simulink model "mcb_param_est_host"  (R2023a)
settings: Solver=FixedStepDiscrete  StartTime=0.0  StopTime=inf  RelTol=1e-3  EnableMultiTasking=on
undefined symbols (not defined in the file): Ts_uart
libraries: instrumentseriallib x3, embeddedblockslib x1, simulink x1
settings Model: Creator=The MathWorks, Inc.  LastModifiedBy=snarayan
settings SolverCC: AlgebraicLoopSolver=TrustRegion
settings DataIOCC: LimitDataPoints=on  SaveFormat=Array  ReturnWorkspaceOutputs=off
settings OptimizationCC: LifeSpan=1  EfficientTunableParamExpr=on
settings DebuggingCC: MergeDetectMultiDrivingBlocksExec=none  SolverPrmCheckMsg=warning  ParameterPrecisionLossMsg=none  UnconnectedInputMsg=warning  UnconnectedOutputMsg=warning  UnconnectedLineMsg=warning  AllowSymbolicDim=off  PregeneratedLibrarySubsystemCodeDiagnostic=none  SFUnexpectedBacktrackingDiag=warning  SFNoUnconditionalDefaultTransitionDiag=warning  SFExecutionAtInitializationDiag=none  ArithmeticOperatorsInVariantConditions=warning
settings HardwareCC: ProdBitPerPointer=32  ProdLargestAtomicFloat=None  ProdIntDivRoundTo=Undefined  ProdEndianess=Unspecified  ProdWordSize=32  ProdHWDeviceType=32-bit Generic
settings ModelReferenceCC: EnableRefExpFcnMdlSchedulingChecks=on  PropagateSignalLabelsOutOfModel=off
settings SFSimCC: SimUseLocalCustomCode=off  MATLABDynamicMemAlloc=off
settings RTWCC: Description=Real-Time Workshop Embedded Coder  SystemTargetFile=ert.tlc  TemplateMakefile=ert_default_tmf  GenerateReport=on  RTWUseLocalCustomCode=off  IncludeHyperlinkInReport=on  LaunchReport=on  GenerateTraceInfo=on  GenerateTraceReport=on  GenerateTraceReportSl=on  GenerateTraceReportSf=on  GenerateTraceReportEml=on  DLArmComputeVersion=19.05
settings CodeAppCC: IgnoreCustomStorageClasses=off  StateflowObjectComments=on  InternalIdentifier=Classic
settings ERTTargetCC: MultiwordLength=2048  GenerateSampleERTMain=on  ERTCustomFileTemplate=example_file_process.tlc  ConvertIfToSwitch=off  SuppressUnreachableDefaultCases=off
settings ConfigComp: CovMetricSettings=dw  CovSaveCumulativeToWorkspaceVar=on  CovSaveSingleToWorkspaceVar=on  CovExternalEMLEnable=off  CovSFcnEnable=off

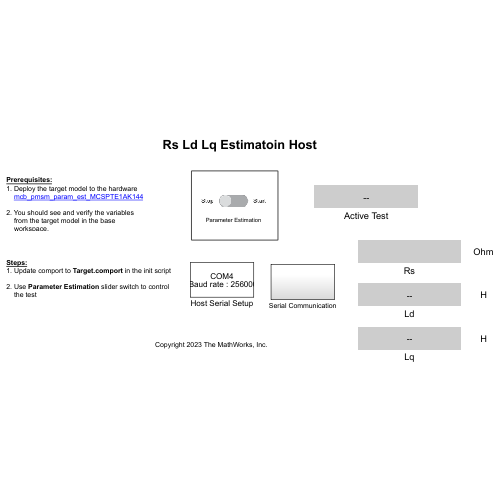
[thumbnail: Simulink's stored preview of the top-level diagram]
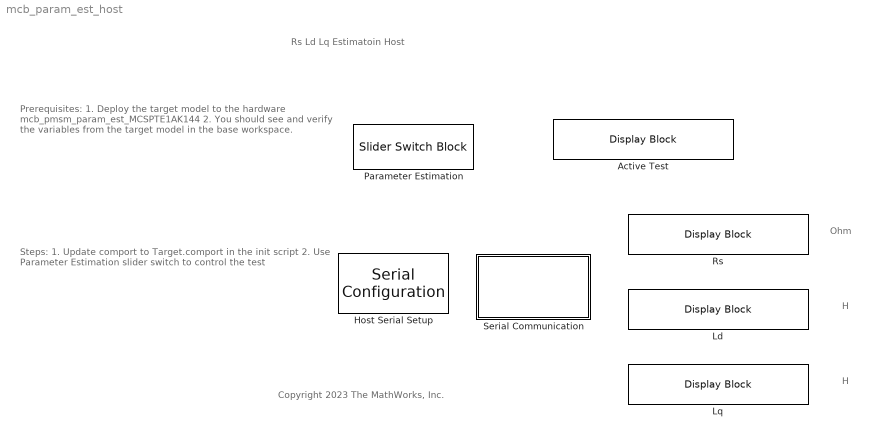
== system mcb_param_est_host ==
  note: Rs Ld Lq Estimatoin Host
  note: Copyright 2023 The MathWorks, Inc.
  note: Ohm
  note: H
  note: H
  note: Prerequisites:
      | 1. Deploy the target model to the hardware
      | mcb_pmsm_param_est_MCSPTE1AK144
      |
      | 2. You should see and verify the variables
      | from the target model in the base
      | workspace.
  note: Steps:
      | 1. Update comport to Target.comport in the init script
      |
      | 2. Use Parameter Estimation slider switch to control
      | the test
  Active Test : DisplayBlock  LabelPosition=Hide  Transparency=1
  Host Serial Setup : instrumentseriallib/Serial Configuration  Priority=-99  PortSel=Target.comport  Port=Target.comport  ComPort=Target.comport  BaudRate=256000  DataBits=8  Parity=none  StopBits=1  ByteOrder=little-endian  FlowControl=none  Timeout=2  SimulateUsing=Interpreted execution  BlockInModel=on  aMode=5
      settings: LibrarySourceBlock=mcbhostblockslib/Host Serial Setup
  Ld : DisplayBlock  LabelPosition=Hide  Transparency=1
  Lq : DisplayBlock  LabelPosition=Hide  Transparency=1
  Parameter Estimation : SliderSwitchBlock  LabelPosition=Hide
      settings: Values={{'Stop', 'Start'}, [0 1]}
  Rs : DisplayBlock  LabelPosition=Hide  Transparency=1
  Serial Communication : Subsystem

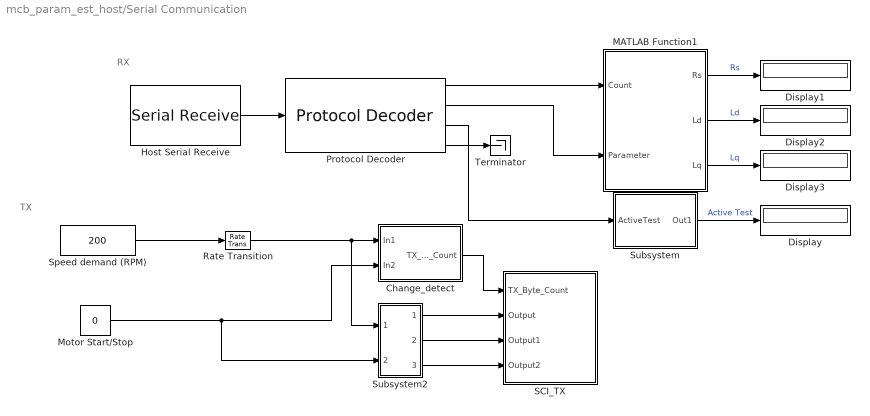
== system mcb_param_est_host/Serial Communication ==
  note: RX
  note: TX
  Change_detect : Subsystem
  Display{,1..3} (4 alike) : Display
  Host Serial Receive : instrumentseriallib/Serial Receive  PortSel=Target.comport  Port=Target.comport  ComPort=Target.comport  DataType=uint8  SaveDataType=uint8  ToggleHeader=off  Header='S'  ToggleTerminator=off  Terminator=Custom terminator  CustomTerminator='E'  InputFormat=Row major  ToggleDataSize=on  DataSize=7  EnableBlockingMode=on  ActionDataUnavailable=Output custom value  ActionWhenDataUnavailable=Output custom value  CustomValue=15  SampleTime=Ts_uart  SimulateUsing=Interpreted execution  BlockInModel=on  aMode=5
      settings: LibrarySourceBlock=mcbhostblockslib/Host Serial Receive
  MATLAB Function1 : MATLAB Function  TreatAsAtomicUnit=on
  Motor Start/Stop : Constant  Value=0  OutDataTypeStr=Inherit: Inherit via back propagation
  Protocol Decoder : embeddedblockslib/Protocol Decoder  IsParseCSV=off  Header='S'  FieldTable={ 'Count', '1', 'uint8', 'Little endian'; 'Parameter', '1', 'single', 'Little endian'; 'Active Test', '1', 'uint8', 'Little endian' }  IsVariableSizeLastField=off  MaxVariableSizeFieldLength=[]  IsChecksumRequired=off  ChecksumAlgorithm=XOR of bytes  ChecksumSize=[]  TerminatorOption=<none>  CustomTerminatorVal=[]  IsInputLengthAvailable=off
      settings: LibrarySourceBlock=c2000lib/Target Communication/Protocol Decoder
  Rate Transition : RateTransition  OutPortSampleTime=Ts_uart
  SCI_TX : Subsystem  TreatAsAtomicUnit=on
  Speed demand (RPM) : Constant  Value=200  VectorParams1D=off  OutDataTypeStr=int16  SampleTime=0.03
  Subsystem : Subsystem
  Subsystem2 : Subsystem
  Terminator : Terminator
  wires:
  Motor Start/Stop/1 -> Subsystem2/2(In2), Change_detect/2(In2)
  Rate Transition/1 -> Subsystem2/1(In1), Change_detect/1(In1)
  Speed demand (RPM)/1 -> Rate Transition/1
  Subsystem2/1(Output) -> SCI_TX/2(Output)
  Subsystem2/2(Output1) -> SCI_TX/3(Output1)
  Subsystem2/3(Output2) -> SCI_TX/4(Output2)
  Change_detect/1(TX_Byte_Count) -> SCI_TX/1(TX_Byte_Count)
  Host Serial Receive/1 -> Protocol Decoder/1
  Protocol Decoder/4 -> Terminator/1
  Protocol Decoder/2 -> MATLAB Function1/2(Parameter)
  MATLAB Function1/1(Rs) -> Display1/1  "Rs"
  MATLAB Function1/2(Ld) -> Display2/1  "Ld"
  MATLAB Function1/3(Lq) -> Display3/1  "Lq"
  Protocol Decoder/1 -> MATLAB Function1/1(Count)
  Protocol Decoder/3 -> Subsystem/1(ActiveTest)
  Subsystem/1(Out1) -> Display/1  "Active Test"

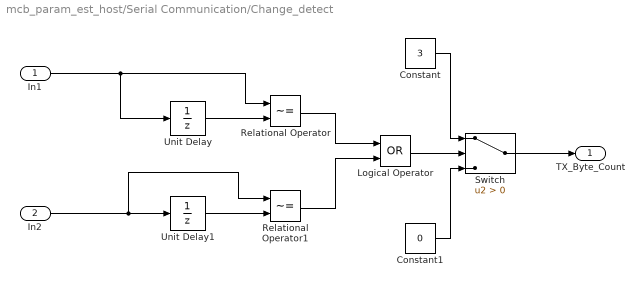
== system mcb_param_est_host/Serial Communication/Change_detect ==
  In1 : Inport
  In2 : Inport  Port=2
  Constant : Constant  Value=3  OutDataTypeStr=uint8
  Constant1 : Constant  Value=0  OutDataTypeStr=uint8
  Logical Operator : Logic  Operator=OR  AllPortsSameDT=off  OutDataTypeStr=boolean
  Relational Operator : RelationalOperator  Operator=~=  OutDataTypeStr=boolean  InputSameDT=off
  Relational Operator1 : RelationalOperator  Operator=~=  OutDataTypeStr=boolean  InputSameDT=off
  Switch : Switch  Criteria=u2 > Threshold  SaturateOnIntegerOverflow=off  InputSameDT=off
  Unit Delay : UnitDelay  InitialCondition=0.5  SampleTime=-1  HasFrameUpgradeWarning=on
  Unit Delay1 : UnitDelay  SampleTime=-1  HasFrameUpgradeWarning=on
  TX_Byte_Count : Outport  VectorParamsAs1DForOutWhenUnconnected=off
  wires:
  In2/1 -> Relational Operator1/1, Unit Delay1/1
  Unit Delay1/1 -> Relational Operator1/2
  Relational Operator1/1 -> Logical Operator/2
  Unit Delay/1 -> Relational Operator/2
  In1/1 -> Relational Operator/1, Unit Delay/1
  Relational Operator/1 -> Logical Operator/1
  Logical Operator/1 -> Switch/2
  Switch/1 -> TX_Byte_Count/1
  Constant/1 -> Switch/1
  Constant1/1 -> Switch/3

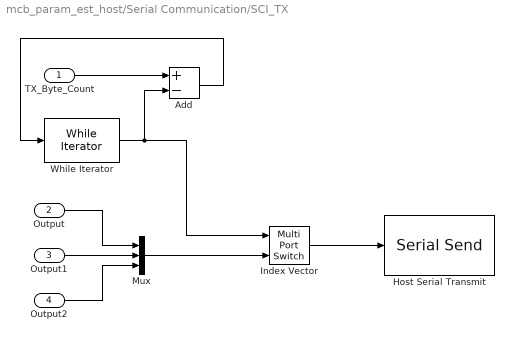
== system mcb_param_est_host/Serial Communication/SCI_TX ==
  TX_Byte_Count : Inport
  Output : Inport  Port=2
  Output1 : Inport  Port=3
  Output2 : Inport  Port=4
  Add : Sum  Inputs=+-  OutDataTypeStr=Inherit: Same as first input
  Host Serial Transmit : instrumentseriallib/Serial Send  PortSel=Target.comport  Port=Target.comport  ComPort=Target.comport  Header=[]  Terminator=<none>  CustomTerminator=[]  EnableBlockingMode=off  SimulateUsing=Interpreted execution  BlockInModel=on  aMode=5
      settings: LibrarySourceBlock=mcbhostblockslib/Host Serial Transmit
  Index Vector : MultiPortSwitch  Inputs=1  SaturateOnIntegerOverflow=off  InputSameDT=off
  Mux : Mux  Inputs=3
  While Iterator : WhileIterator  MaxIters=3  WhileBlockType=do-while  ShowIterationPort=on  OutputDataType=int16
  wires:
  Output/1 -> Mux/1
  Mux/1 -> Index Vector/2
  Output2/1 -> Mux/3
  Add/1 -> While Iterator/1
  Output1/1 -> Mux/2
  TX_Byte_Count/1 -> Add/1
  While Iterator/1 -> Index Vector/1, Add/2
  Index Vector/1 -> Host Serial Transmit/1

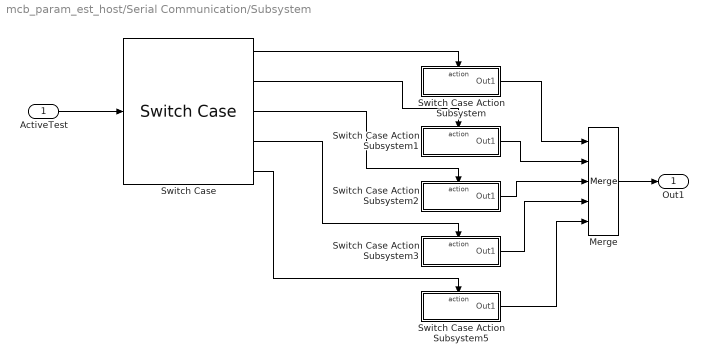
== system mcb_param_est_host/Serial Communication/Subsystem ==
  ActiveTest : Inport
  Merge : Merge  Inputs=5
  Switch Case : SwitchCase  CaseConditions={0,1,2,3}
  Switch Case Action Subsystem : Subsystem  TreatAsAtomicUnit=on
  Switch Case Action Subsystem1 : Subsystem  TreatAsAtomicUnit=on
  Switch Case Action Subsystem2 : Subsystem  TreatAsAtomicUnit=on
  Switch Case Action Subsystem3 : Subsystem  TreatAsAtomicUnit=on
  Switch Case Action Subsystem5 : Subsystem  TreatAsAtomicUnit=on
  Out1 : Outport
  wires:
  Merge/1 -> Out1/1
  ActiveTest/1 -> Switch Case/1
  Switch Case/1 -> Switch Case Action Subsystem/Action
  Switch Case/2 -> Switch Case Action Subsystem1/Action
  Switch Case/3 -> Switch Case Action Subsystem2/Action
  Switch Case/4 -> Switch Case Action Subsystem3/Action
  Switch Case/5 -> Switch Case Action Subsystem5/Action
  Switch Case Action Subsystem1/1(Out1) -> Merge/2
  Switch Case Action Subsystem2/1(Out1) -> Merge/3
  Switch Case Action Subsystem/1(Out1) -> Merge/1
  Switch Case Action Subsystem3/1(Out1) -> Merge/4
  Switch Case Action Subsystem5/1(Out1) -> Merge/5

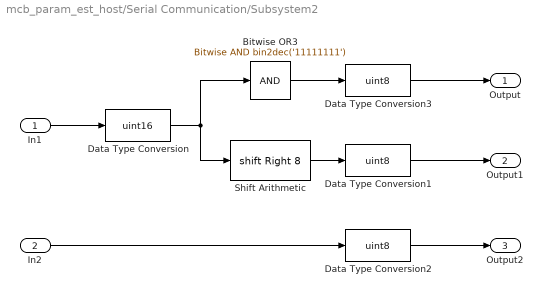
== system mcb_param_est_host/Serial Communication/Subsystem2 ==
  In1 : Inport
  In2 : Inport  Port=2
  Bitwise OR3 : simulink/Logic and Bit Operations/Bitwise Operator  logicop=AND  UseBitMask=on  BitMask=bin2dec('11111111')  BitMaskRealWorld=Stored Integer
  Data Type Conversion : DataTypeConversion  OutDataTypeStr=uint16  ConvertRealWorld=Stored Integer (SI)  RndMeth=Simplest  SaturateOnIntegerOverflow=off
  Data Type Conversion1 : DataTypeConversion  OutDataTypeStr=uint8  ConvertRealWorld=Stored Integer (SI)  RndMeth=Simplest  SaturateOnIntegerOverflow=off
  Data Type Conversion2 : DataTypeConversion  OutDataTypeStr=uint8  ConvertRealWorld=Stored Integer (SI)  RndMeth=Simplest  SaturateOnIntegerOverflow=off
  Data Type Conversion3 : DataTypeConversion  OutDataTypeStr=uint8  ConvertRealWorld=Stored Integer (SI)  RndMeth=Simplest  SaturateOnIntegerOverflow=off
  Shift Arithmetic : ArithShift  BitShiftNumber=8  BitShiftDirection=Right
  Output : Outport
  Output1 : Outport  Port=2
  Output2 : Outport  Port=3
  wires:
  Data Type Conversion2/1 -> Output2/1
  Data Type Conversion/1 -> Bitwise OR3/1, Shift Arithmetic/1
  In1/1 -> Data Type Conversion/1
  Bitwise OR3/1 -> Data Type Conversion3/1
  Shift Arithmetic/1 -> Data Type Conversion1/1
  In2/1 -> Data Type Conversion2/1
  Data Type Conversion1/1 -> Output1/1
  Data Type Conversion3/1 -> Output/1

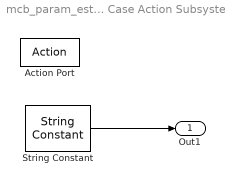
== system mcb_param_est_host/Serial Communication/Subsystem/Switch Case Action Subsystem ==
  Action Port : ActionPort
  String Constant : StringConstant  String="\"Inactive\""
  Out1 : Outport
  wires:
  String Constant/1 -> Out1/1

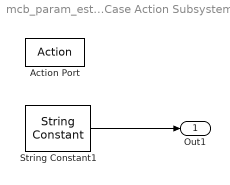
== system mcb_param_est_host/Serial Communication/Subsystem/Switch Case Action Subsystem1 ==
  Action Port : ActionPort
  String Constant1 : StringConstant  String="\"Rs Test\""
  Out1 : Outport
  wires:
  String Constant1/1 -> Out1/1

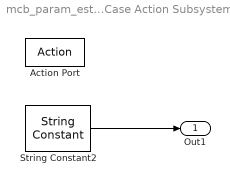
== system mcb_param_est_host/Serial Communication/Subsystem/Switch Case Action Subsystem2 ==
  Action Port : ActionPort
  String Constant2 : StringConstant  String="\"Ld Test\""
  Out1 : Outport
  wires:
  String Constant2/1 -> Out1/1

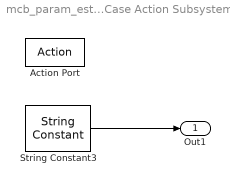
== system mcb_param_est_host/Serial Communication/Subsystem/Switch Case Action Subsystem3 ==
  Action Port : ActionPort
  String Constant3 : StringConstant  String="\"Lq Test\""
  Out1 : Outport
  wires:
  String Constant3/1 -> Out1/1

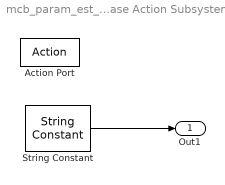
== system mcb_param_est_host/Serial Communication/Subsystem/Switch Case Action Subsystem5 ==
  Action Port : ActionPort
  String Constant : StringConstant  String="\"Inactive\""
  Out1 : Outport
  wires:
  String Constant/1 -> Out1/1

== matlab function mcb_param_est_host/Serial Communication/MATLAB Function1 ==
  data: Rs output; Ld output; Lq output; Count input; Parameter input
function [ Rs, Ld, Lq] = unBuf(Count, Parameter)

coder.extrinsic('message', 'msgbox', 'set_param', 'error');

persistent RsLocal;             % To count the number of Id samples
if isempty(RsLocal)
	RsLocal = single(0);
end

persistent LdLocal;             % To count the number of Id samples
if isempty(LdLocal)
	LdLocal = single(0);
end

persistent LqLocal;             % To count the number of Id samples
if isempty(LqLocal)
	LqLocal = single(0);
end

if (Count == 1 )
    RsLocal = Parameter;
elseif (Count == 2 )
    LdLocal = Parameter;
elseif (Count == 3 )
    LqLocal = Parameter;
end

Rs = RsLocal;
Ld = LdLocal;
Lq = LqLocal;

end
